simulink model "MSD_Estimate"  (R2025b)
settings: Solver=FixedStepAuto  StartTime=0.0  StopTime=60  FixedStep=0.001  RelTol=1e-3
values from neighbouring files (symbols this model uses):
  F = [1 dt ... (first row only)    [KalmanFilter.m]
undefined symbols (not defined in the file or in its folder): k, m, x_inti
settings Model: Creator=Akkarasaknarong  LastModifiedBy=Akkarasaknarong

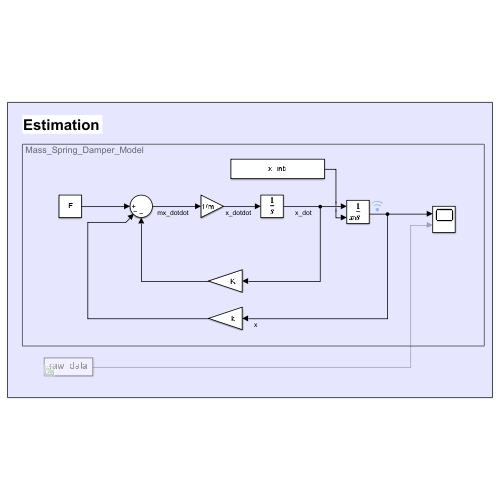
[thumbnail: Simulink's stored preview of the top-level diagram]
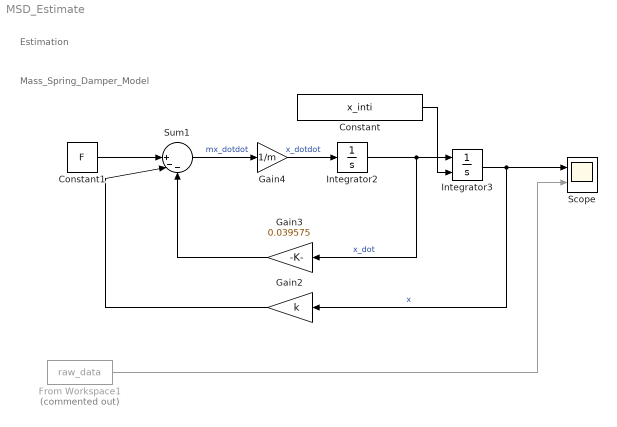
== system MSD_Estimate ==
  note: Mass_Spring_Damper_Model
  note: Estimation
  Constant : Constant  Value=x_inti
  Constant1 : Constant  Value=F
  From Workspace1 : FromWorkspace  Commented=on  VariableName=raw_data
  Gain2 : Gain  Gain=k
  Gain3 : Gain  Gain=0.039575
  Gain4 : Gain  Gain=1/m
  Integrator2 : Integrator
  Integrator3 : Integrator  InitialConditionSource=external
  Scope : Scope  NumInputPorts=2
      settings: ActiveDisplayYMinimum=-0.083681997318588816  ActiveDisplayYMaximum=0.082448358466179386
  Sum1 : Sum  Inputs=||+--
  wires:
  Constant1/1 -> Sum1/1
  Gain4/1 -> Integrator2/1  "x_dotdot"
  Gain2/1 -> Sum1/2
  Sum1/1 -> Gain4/1  "mx_dotdot"
  Integrator3/1 -> Gain2/1, Scope/1  "x"
  Integrator2/1 -> Gain3/1, Integrator3/1  "x_dot"
  Gain3/1 -> Sum1/3
  Constant/1 -> Integrator3/2
  From Workspace1/1 -> Scope/2
